simulink model "ModeloManual"  (R2022a)
settings: Solver=VariableStepAuto  StartTime=0.0  StopTime=10  RelTol=1e-3
values from neighbouring files (symbols this model uses):
  a = 0.2    [Data.m]
  alturaobst = 0.9    [Data.m]
  b = 0.542    [Data.m]
  M = [x_new y_new]    [Data.m]
  M_chasis = 3    [Data.m]
  M_rueda = 1    [Data.m]
  M_ruedacontacto = 1    [Data.m]
  N = 4365    [GraficasVelocidades.m]    (also in Prueba_Liapunov.m = length(p_X); WaypointsToTrayectory.m = length(X))
  R = 0.175/2    (= 0.0875)    [Data.m]
  X = M(:,1)    [WaypointsToTrayectory.m]
  x0 = x_ini(1)*factorE    [Data.m]
  x_obj = pos_fin(1)*factorE    [Data.m]
  xobstac = RandomPos(1)    [Data.m]
  Y = M(:, 2)    [WaypointsToTrayectory.m]
  y0 = y_ini(2)*factorE    [Data.m]
  y_obj = pos_fin(2)*factorE    [Data.m]
  yobstac = RandomPos(2)    [Data.m]
  zobstac = RandomPos(3)    [Data.m]
undefined symbols (not defined in the file or in its folder): bloqueobstaculo, Borde11, Borde12, Borde2, Borde3, Borde41, Borde42, Explanada, plano150g1, plano150g2, plano150g3, plano150g4, Plano150mm, plano150mm2irr, Plano45mm, plano45mm2irr, Plano90mm, Rampa, Rampa21, Rampa22, Rampa31, Rampa32, Rampa33, Rampa4, Rampa51, Rampa52, Rampa53, Terreno, Z
libraries: sm_lib x331, nesl_utility x30, fl_lib x3, robotalgslib x1
(part 5 of 8)

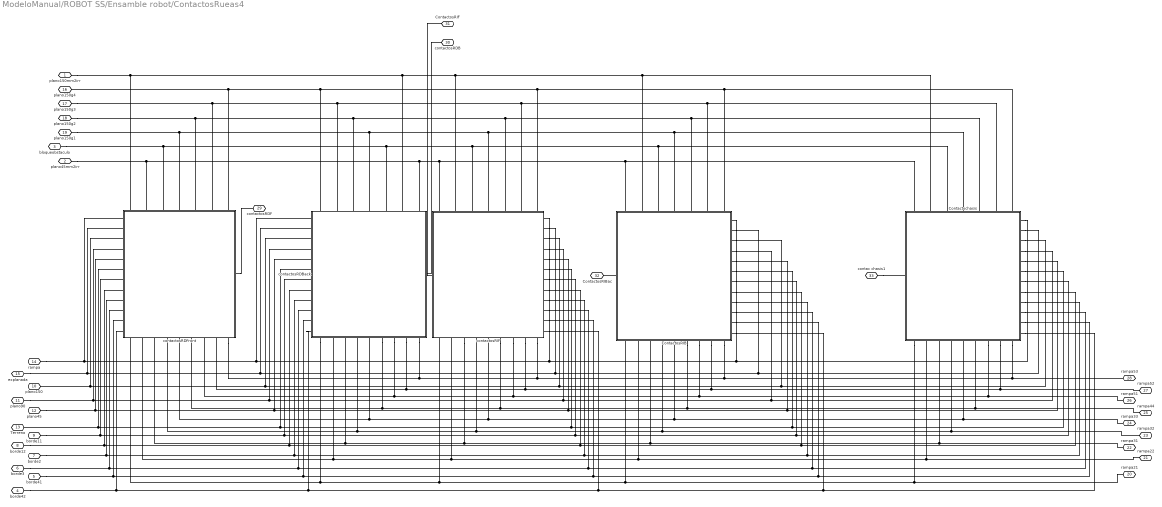
== system ModeloManual/ROBOT SS/Ensamble robot/ContactosRueas4 ==
  Contactochasis : Subsystem
      settings: PortSchema="{\"entries\":[{\"content\":{\"sides\":[{\"content\":{\"connectorIds\":[\"LConn1\"]},\"type\":\"ConnectorPlacement.EquallySpacedRectSide\",\"uuid\":\"4f581815-8ae4-4ee7-9b05-a8dd2e10ae63\"},{\"content\":{\"connectorIds\":[\"RConn1\",\"RConn2\",\"RConn3\",\"RConn4\",\"RConn5\",\"RConn6\",\"RConn7\",\"RConn8\",\"RConn9\",\"RConn10\",\"RConn11\",\"RConn12\"],\"side\":\"RIGHT\"},\"type\":\"ConnectorPlacement.EquallySpacedRectSide\",\"uuid\":\"8325c4e1-14be-4d51-94f3-53093c654f2d\"},{\"content\":{\"connectorIds\":[\"LConn2\",\"LConn3\",\"LConn4\",\"LConn5\",\"LConn6\",\"LConn7\",\"LConn8\",\"LConn9\",\"LConn10\"],\"side\":\"TOP\"},\"type\":\"ConnectorPlacement.EquallySpacedRectSide\",\"uuid\":\"45878acc-deff-4729-a66d-73775d7e8d0b\"},{\"content\":{\"connectorIds\":[\"RConn13\",\"RConn14\",\"RConn15\",\"RConn16\",\"RConn17\",\"RConn18\",\"RConn19\"],\"side\":\"BOTTOM\"},\"type\":\"ConnectorPlacement.EquallySpacedRectSide\",\"uuid\":\"dca1d019-3cd3-4a64-96c4-a5ef2847eb3c\"}]},\"type\":\"ConnectorPlacement.EquallySpacedConnector\",\"uuid\":\"5432a14d-752f-4214-bad7-a9a48797e409\"}],\"packageUris\":[\"http://schema.mathworks.com/mf0/Connector/R2020b\"],\"version\":\"1.0\"}"
  ContactosRIB : Subsystem
      settings: PortSchema="{\"entries\":[{\"content\":{\"sides\":[{\"content\":{\"connectorIds\":[\"LConn1\"]},\"type\":\"ConnectorPlacement.EquallySpacedRectSide\",\"uuid\":\"4f581815-8ae4-4ee7-9b05-a8dd2e10ae63\"},{\"content\":{\"connectorIds\":[\"RConn1\",\"RConn2\",\"RConn3\",\"RConn4\",\"RConn5\",\"RConn6\",\"RConn7\",\"RConn8\",\"RConn9\",\"RConn10\",\"RConn11\",\"RConn12\"],\"side\":\"RIGHT\"},\"type\":\"ConnectorPlacement.EquallySpacedRectSide\",\"uuid\":\"8325c4e1-14be-4d51-94f3-53093c654f2d\"},{\"content\":{\"connectorIds\":[\"LConn2\",\"LConn3\",\"LConn4\",\"LConn5\",\"LConn6\",\"LConn7\",\"LConn8\",\"LConn9\",\"LConn10\"],\"side\":\"TOP\"},\"type\":\"ConnectorPlacement.EquallySpacedRectSide\",\"uuid\":\"45878acc-deff-4729-a66d-73775d7e8d0b\"},{\"content\":{\"connectorIds\":[\"RConn13\",\"RConn14\",\"RConn15\",\"RConn16\",\"RConn17\",\"RConn18\",\"RConn19\"],\"side\":\"BOTTOM\"},\"type\":\"ConnectorPlacement.EquallySpacedRectSide\",\"uuid\":\"dca1d019-3cd3-4a64-96c4-a5ef2847eb3c\"}]},\"type\":\"ConnectorPlacement.EquallySpacedConnector\",\"uuid\":\"5432a14d-752f-4214-bad7-a9a48797e409\"}],\"packageUris\":[\"http://schema.mathworks.com/mf0/Connector/R2020b\"],\"version\":\"1.0\"}"
  contactosRDBack : Subsystem
      settings: PortSchema="{\"entries\":[{\"content\":{\"sides\":[{\"content\":{\"connectorIds\":[\"LConn1\",\"LConn2\",\"LConn3\",\"LConn4\",\"LConn5\",\"LConn6\",\"LConn7\",\"LConn8\",\"LConn9\",\"LConn10\",\"LConn11\",\"LConn12\"]},\"type\":\"ConnectorPlacement.EquallySpacedRectSide\",\"uuid\":\"4677d3c0-fe6b-4e84-8f73-c854d9b35b96\"},{\"content\":{\"connectorIds\":[\"RConn1\"],\"side\":\"RIGHT\"},\"type\":\"ConnectorPlacement.EquallySpacedRectSide\",\"uuid\":\"c55e0516-1ae0-4a26-a435-c2ac17281f56\"},{\"content\":{\"connectorIds\":[\"LConn13\",\"LConn14\",\"LConn15\",\"LConn16\",\"LConn17\",\"LConn18\",\"LConn19\",\"LConn20\",\"LConn21\"],\"side\":\"TOP\"},\"type\":\"ConnectorPlacement.EquallySpacedRectSide\",\"uuid\":\"54ab0c51-bb18-4865-8b25-0e77e88e8b63\"},{\"content\":{\"connectorIds\":[\"RConn2\",\"RConn3\",\"RConn4\",\"RConn5\",\"RConn6\",\"RConn7\",\"RConn8\"],\"side\":\"BOTTOM\"},\"type\":\"ConnectorPlacement.EquallySpacedRectSide\",\"uuid\":\"810dc9ff-bd8f-4485-b930-6348a4343a1c\"}]},\"type\":\"ConnectorPlacement.EquallySpacedConnector\",\"uuid\":\"c5f80127-49af-43c5-b6ef-5a46cea3903d\"}],\"packageUris\":[\"http://schema.mathworks.com/mf0/Connector/R2020b\"],\"version\":\"1.0\"}"
  contactosRDFront : Subsystem
      settings: PortSchema="{\"entries\":[{\"content\":{\"sides\":[{\"content\":{\"connectorIds\":[\"LConn1\",\"LConn2\",\"LConn3\",\"LConn4\",\"LConn5\",\"LConn6\",\"LConn7\",\"LConn8\",\"LConn9\",\"LConn10\",\"LConn11\",\"LConn12\"]},\"type\":\"ConnectorPlacement.EquallySpacedRectSide\",\"uuid\":\"4677d3c0-fe6b-4e84-8f73-c854d9b35b96\"},{\"content\":{\"connectorIds\":[\"RConn1\"],\"side\":\"RIGHT\"},\"type\":\"ConnectorPlacement.EquallySpacedRectSide\",\"uuid\":\"c55e0516-1ae0-4a26-a435-c2ac17281f56\"},{\"content\":{\"connectorIds\":[\"LConn13\",\"LConn14\",\"LConn15\",\"LConn16\",\"LConn17\",\"LConn18\",\"LConn19\",\"LConn20\",\"LConn21\"],\"side\":\"TOP\"},\"type\":\"ConnectorPlacement.EquallySpacedRectSide\",\"uuid\":\"54ab0c51-bb18-4865-8b25-0e77e88e8b63\"},{\"content\":{\"connectorIds\":[\"RConn2\",\"RConn3\",\"RConn4\",\"RConn5\",\"RConn6\",\"RConn7\",\"RConn8\"],\"side\":\"BOTTOM\"},\"type\":\"ConnectorPlacement.EquallySpacedRectSide\",\"uuid\":\"1e9ef993-c1dc-4ae7-9992-9b6ea278c652\"}]},\"type\":\"ConnectorPlacement.EquallySpacedConnector\",\"uuid\":\"c5f80127-49af-43c5-b6ef-5a46cea3903d\"}],\"packageUris\":[\"http://schema.mathworks.com/mf0/Connector/R2020b\"],\"version\":\"1.0\"}"
  contactosRIF : Subsystem
      settings: PortSchema="{\"entries\":[{\"content\":{\"sides\":[{\"content\":{\"connectorIds\":[\"LConn1\"]},\"type\":\"ConnectorPlacement.EquallySpacedRectSide\",\"uuid\":\"4f581815-8ae4-4ee7-9b05-a8dd2e10ae63\"},{\"content\":{\"connectorIds\":[\"RConn1\",\"RConn2\",\"RConn3\",\"RConn4\",\"RConn5\",\"RConn6\",\"RConn7\",\"RConn8\",\"RConn9\",\"RConn10\",\"RConn11\",\"RConn12\"],\"side\":\"RIGHT\"},\"type\":\"ConnectorPlacement.EquallySpacedRectSide\",\"uuid\":\"8325c4e1-14be-4d51-94f3-53093c654f2d\"},{\"content\":{\"connectorIds\":[\"LConn2\",\"LConn3\",\"LConn4\",\"LConn5\",\"LConn6\",\"LConn7\",\"LConn8\",\"LConn9\",\"LConn10\"],\"side\":\"TOP\"},\"type\":\"ConnectorPlacement.EquallySpacedRectSide\",\"uuid\":\"45878acc-deff-4729-a66d-73775d7e8d0b\"},{\"content\":{\"connectorIds\":[\"RConn13\",\"RConn14\",\"RConn15\",\"RConn16\",\"RConn17\",\"RConn18\",\"RConn19\"],\"side\":\"BOTTOM\"},\"type\":\"ConnectorPlacement.EquallySpacedRectSide\",\"uuid\":\"4d447f89-609c-4778-adb6-6019672adf15\"}]},\"type\":\"ConnectorPlacement.EquallySpacedConnector\",\"uuid\":\"5432a14d-752f-4214-bad7-a9a48797e409\"}],\"packageUris\":[\"http://schema.mathworks.com/mf0/Connector/R2020b\"],\"version\":\"1.0\"}"
  plano150mm2irr : PMIOPort  Side=Left
  plano45mm2irr : PMIOPort  Port=2  Side=Left
  bloqueobstaculo : PMIOPort  Port=3  Side=Left
  borde42 : PMIOPort  Port=4  Side=Left
  borde41 : PMIOPort  Port=5  Side=Left
  borde3 : PMIOPort  Port=6  Side=Left
  borde2 : PMIOPort  Port=7  Side=Left
  borde12 : PMIOPort  Port=8  Side=Left
  borde11 : PMIOPort  Port=9  Side=Left
  plano150 : PMIOPort  Port=10  Side=Left
  plano90 : PMIOPort  Port=11  Side=Left
  plano45 : PMIOPort  Port=12  Side=Left
  Terreno : PMIOPort  Port=13  Side=Left
  rampa : PMIOPort  Port=14  Side=Left
  explanada : PMIOPort  Port=15  Side=Left
  plano150g4 : PMIOPort  Port=16  Side=Left
  plano150g3 : PMIOPort  Port=17  Side=Left
  plano150g2 : PMIOPort  Port=18  Side=Left
  plano150g1 : PMIOPort  Port=19  Side=Left
  rampa21 : PMIOPort  Port=20  Side=Left
  rampa22 : PMIOPort  Port=21  Side=Left
  rampa31 : PMIOPort  Port=22  Side=Left
  rampa32 : PMIOPort  Port=23  Side=Left
  rampa33 : PMIOPort  Port=24  Side=Left
  rampa44 : PMIOPort  Port=25  Side=Left
  rampa51 : PMIOPort  Port=26  Side=Left
  rampa52 : PMIOPort  Port=27  Side=Left
  rampa53 : PMIOPort  Port=28  Side=Left
  contactosRDF : PMIOPort  Port=29  Side=Right
  contactosRDB : PMIOPort  Port=30  Side=Right
  ContactosRIF : PMIOPort  Port=31  Side=Right
  ContactosRIBac : PMIOPort  Port=32  Side=Right
  contac chasis1 : PMIOPort  Port=33  Side=Right
  connections:
  plano45/RConn1 -- Contactochasis/RConn8 -- ContactosRIB/RConn8 -- contactosRIF/RConn8 -- contactosRDBack/LConn8 -- contactosRDFront/LConn8
  contactosRDFront/LConn7 -- Contactochasis/RConn7 -- ContactosRIB/RConn7 -- contactosRIF/RConn7 -- contactosRDBack/LConn7 -- Terreno/RConn1
  contactosRDFront/RConn1 -- contactosRDF/RConn1
  contactosRDBack/RConn1 -- contactosRDB/RConn1
  plano90/RConn1 -- Contactochasis/RConn9 -- ContactosRIB/RConn9 -- contactosRIF/RConn9 -- contactosRDBack/LConn9 -- contactosRDFront/LConn9
  explanada/RConn1 -- Contactochasis/RConn11 -- ContactosRIB/RConn11 -- contactosRIF/RConn11 -- contactosRDBack/LConn11 -- contactosRDFront/LConn11
  rampa/RConn1 -- Contactochasis/RConn12 -- ContactosRIB/RConn12 -- contactosRIF/RConn12 -- contactosRDBack/LConn12 -- contactosRDFront/LConn12
  contactosRDFront/LConn10 -- Contactochasis/RConn10 -- ContactosRIB/RConn10 -- contactosRIF/RConn10 -- contactosRDBack/LConn10 -- plano150/RConn1
  ContactosRIF/RConn1 -- contactosRIF/LConn1
  ContactosRIB/LConn1 -- ContactosRIBac/RConn1
  borde11/RConn1 -- Contactochasis/RConn6 -- ContactosRIB/RConn6 -- contactosRIF/RConn6 -- contactosRDBack/LConn6 -- contactosRDFront/LConn6
  borde12/RConn1 -- Contactochasis/RConn5 -- ContactosRIB/RConn5 -- contactosRIF/RConn5 -- contactosRDBack/LConn5 -- contactosRDFront/LConn5
  borde2/RConn1 -- ContactosRIB/RConn4 -- Contactochasis/RConn4 -- contactosRIF/RConn4 -- contactosRDBack/LConn4 -- contactosRDFront/LConn4
  borde3/RConn1 -- Contactochasis/RConn3 -- ContactosRIB/RConn3 -- contactosRIF/RConn3 -- contactosRDBack/LConn3 -- contactosRDFront/LConn3
  borde41/RConn1 -- Contactochasis/RConn2 -- ContactosRIB/RConn2 -- contactosRIF/RConn2 -- contactosRDBack/LConn2 -- contactosRDFront/LConn2
  borde42/RConn1 -- Contactochasis/RConn1 -- ContactosRIB/RConn1 -- contactosRIF/RConn1 -- contactosRDBack/LConn1 -- contactosRDFront/LConn1
  contactosRDFront/LConn21 -- contactosRDBack/LConn21 -- contactosRIF/LConn10 -- ContactosRIB/LConn10 -- rampa53/RConn1 -- Contactochasis/LConn10
  rampa52/RConn1 -- Contactochasis/LConn9 -- ContactosRIB/LConn9 -- contactosRIF/LConn9 -- contactosRDBack/LConn20 -- contactosRDFront/LConn20
  rampa51/RConn1 -- Contactochasis/LConn8 -- ContactosRIB/LConn8 -- contactosRIF/LConn8 -- contactosRDBack/LConn19 -- contactosRDFront/LConn19
  rampa44/RConn1 -- Contactochasis/LConn7 -- ContactosRIB/LConn7 -- contactosRIF/LConn7 -- contactosRDBack/LConn18 -- contactosRDFront/LConn18
  rampa33/RConn1 -- Contactochasis/LConn6 -- ContactosRIB/LConn6 -- contactosRIF/LConn6 -- contactosRDBack/LConn17 -- contactosRDFront/LConn17
  rampa32/RConn1 -- Contactochasis/LConn5 -- ContactosRIB/LConn5 -- contactosRIF/LConn5 -- contactosRDBack/LConn16 -- contactosRDFront/LConn16
  rampa31/RConn1 -- Contactochasis/LConn4 -- ContactosRIB/LConn4 -- contactosRIF/LConn4 -- contactosRDBack/LConn15 -- contactosRDFront/LConn15
  rampa22/RConn1 -- Contactochasis/LConn3 -- ContactosRIB/LConn3 -- contactosRIF/LConn3 -- contactosRDBack/LConn14 -- contactosRDFront/LConn14
  rampa21/RConn1 -- ContactosRIB/LConn2 -- contactosRIF/LConn2 -- contactosRDBack/LConn13 -- contactosRDFront/LConn13 -- Contactochasis/LConn2
  contac chasis1/RConn1 -- Contactochasis/LConn1
  Contactochasis/RConn19 -- contactosRIF/RConn19 -- contactosRDFront/RConn8 -- plano150g4/RConn1 -- contactosRDBack/RConn2 -- ContactosRIB/RConn19
  plano150g3/RConn1 -- contactosRIF/RConn18 -- ContactosRIB/RConn18 -- Contactochasis/RConn18 -- contactosRDBack/RConn3 -- contactosRDFront/RConn7
  plano150g2/RConn1 -- contactosRDFront/RConn6 -- contactosRDBack/RConn4 -- contactosRIF/RConn17 -- Contactochasis/RConn17 -- ContactosRIB/RConn17
  plano150g1/RConn1 -- contactosRIF/RConn16 -- ContactosRIB/RConn16 -- Contactochasis/RConn16 -- contactosRDBack/RConn5 -- contactosRDFront/RConn5
  bloqueobstaculo/RConn1 -- contactosRDBack/RConn6 -- contactosRIF/RConn15 -- ContactosRIB/RConn15 -- Contactochasis/RConn15 -- contactosRDFront/RConn4
  plano150mm2irr/RConn1 -- contactosRIF/RConn14 -- ContactosRIB/RConn14 -- Contactochasis/RConn14 -- contactosRDBack/RConn7 -- contactosRDFront/RConn2
  plano45mm2irr/RConn1 -- ContactosRIB/RConn13 -- Contactochasis/RConn13 -- contactosRIF/RConn13 -- contactosRDBack/RConn8 -- contactosRDFront/RConn3

== system ModeloManual/ROBOT SS/Ensamble robot/RDBack ==
  Cylindrical Solid : sm_lib/Body Elements/Cylindrical Solid  GraphicAmbientColor=[0.15 0.15 0.15 1.0]  BasedOnType=Mass  CenterOfMass=[0 0 0]  CenterOfMassUnits=m  GraphicDiffuseColor=[1.0 0.0 0.2]  CylinderLength=0.045  CylinderLengthUnits=m  CylinderRadius=0.0826  CylinderRadiusUnits=m  Density=1000  DensityUnits=kg/m^3  DoExposeReferenceFrame=on  GraphicEmissiveColor=[0.0 0.0 0.0 1.0]  ExportEntireGeometry=on  SerializedFrames=<Frames/>  MarkerShape=Sphere  MarkerSize=10  GraphicType=None  InertiaType=CalculateFromGeometry  Mass=M_ruedacontacto  MassUnits=kg  MomentsOfInertia=[1 1 1]  MomentsOfInertiaUnits=kg*m^2  GraphicOpacity=1.0  ProductsOfInertia=[0 0 0]  ProductsOfInertiaUnits=kg*m^2  GraphicShininess=75  GraphicSpecularColor=[0.5 0.5 0.5 1.0]  GraphicVisPropType=SimpleVisualProperties
  PS-Simulink Converter : nesl_utility/PS-Simulink Converter  PhysicalDomain=network_engine_domain  SubClassName=ps_output  LeftPortType=input  RightPortType=output  PseudoPeriodic=off  Frequencies=[]  VectorFormat=inherit  Unit=inherit  AffineConversion=off
      settings: SourceProductBaseCode=SS,PW,VE
  Revolute Joint1 : sm_lib/Joints/Revolute Joint  JointMode=Normal  SenseConstraintForce=off  SenseConstraintForceX=off  SenseConstraintForceY=off  SenseConstraintForceZ=off  SenseConstraintTorque=off  SenseConstraintTorqueX=off  SenseConstraintTorqueY=off  SenseConstraintTorqueZ=off  SenseTotalForce=off  SenseTotalForceX=off  SenseTotalForceY=off  SenseTotalForceZ=off  SenseTotalTorque=off  SenseTotalTorqueX=off  SenseTotalTorqueY=off  SenseTotalTorqueZ=off  CompositeWrenchDir=FollowerOnBase  CompositeWrenchFrame=BaseFrame  EquilibriumPosition=0  EquilibriumPositionUnits=rad  SpringStiffness=0  SpringStiffnessUnits=N*m/rad  DampingCoefficient=0  DampingCoefficientUnits=N*m/(rad/s)  TorqueActuationMode=ComputedTorque  MotionActuationMode=InputMotion  SensePosition=off  SenseVelocity=on  SenseAcceleration=off  SenseTorqueForce=off  SenseLowerLimitTorqueForce=off  SenseUpperLimitTorqueForce=off  LowerLimitSpecify=off  LowerLimitBound=-90  LowerLimitBoundUnits=deg  LowerLimitStiffness=1e4  LowerLimitStiffnessUnits=N*m/deg  LowerLimitDamping=10  LowerLimitDampingUnits=N*m/(deg/s)  LowerLimitTransitionRegionWidth=0.1  LowerLimitTransitionRegionWidthUnits=deg  UpperLimitSpecify=off  UpperLimitBound=90  UpperLimitBoundUnits=deg  UpperLimitStiffness=1e4  UpperLimitStiffnessUnits=N*m/deg  UpperLimitDamping=10  UpperLimitDampingUnits=N*m/(deg/s)  UpperLimitTransitionRegionWidth=0.1  UpperLimitTransitionRegionWidthUnits=deg  PositionTargetSpecify=off  PositionTargetPriority=High  PositionTargetValue=0  PositionTargetValueUnits=deg  VelocityTargetSpecify=off  VelocityTargetPriority=High  VelocityTargetValue=0  VelocityTargetValueUnits=deg/s
  Rigid Transform1 : sm_lib/Frames and Transforms/Rigid Transform  TranslationMethod=None  TranslationStandardOffset=10  TranslationLengthUnit=mm  TranslationStandardAxis=-X  TranslationCartesianOffset=[0 0 0]  TranslationROffset=0  TranslationROffsetUnits=m  TranslationZOffset=0  TranslationZOffsetUnits=m  TranslationThetaOffset=0  TranslationThetaOffsetUnits=deg  RotationMethod=StandardAxis  RotationAngleUnits=deg  RotationStandardAxis=-Y  RotationAngle=90  RotationArbitraryAxis=[0 0 1]  FollAlignAxisA=+X  BaseAlignAxisA=+Y  FollAlignAxisB=+Y  BaseAlignAxisB=+Z  RotationSequenceAxes=FollowerAxes  RotationSequence=XYZ  RotationSequenceAngles=[0 0 0]  RotationSequenceAnglesUnits=deg  RotationMatrix=[1 0 0; 0 1 0; 0 0 1]
  Rueda1 : sm_lib/Body Elements/File Solid  ExtGeomFileName=rueda_nueva_contodo.stp  UnitType=FromFile  ExtGeomFileUnits=m  StepReaderType=HEX  ExportConvexHullGeometry=off  InertiaType=CalculateFromGeometry  Mass=M_rueda  MassUnits=kg  CenterOfMass=[0 0 0]  CenterOfMassUnits=m  MomentsOfInertia=[1 1 1]  MomentsOfInertiaUnits=kg*m^2  ProductsOfInertia=[0 0 0]  ProductsOfInertiaUnits=kg*m^2  BasedOnType=Density  Density=D_rueda  DensityUnits=kg/m^3  DoExposeReferenceFrame=on  SerializedFrames=<Frames><Frame><Id>Frame1</Id><Value><Name>F1</Name><Origin><Source>CenterOfMassFrame</Source><FeatureName></FeatureName></Origin><PrimaryAxis><DefinedDirection>+X</DefinedDirection><Source>ReferenceFrame</Source><SourceDirection>+Z</SourceDirection><FeatureName></FeatureName></PrimaryAxis><SecondaryAxis><DefinedDirection>-Z</DefinedDirection><Source>ReferenceFrame</Source><SourceDirection>+X</SourceDirection><FeatureName></FeatureName></SecondaryAxis></Value></Frame></Frames>  GraphicType=FromGeometry  MarkerShape=Sphere  MarkerSize=10  GraphicVisPropType=SimpleVisualProperties  GraphicDiffuseColor=[0 0 0]  GraphicSpecularColor=[0.5 0.5 0.5 1.0]  GraphicAmbientColor=[0.15 0.15 0.15 1.0]  GraphicEmissiveColor=[0.0 0.0 0.0 1.0]  GraphicShininess=75  GraphicOpacity=1.0
  W2 : PMIOPort  Side=Left
  F : PMIOPort  Port=2  Side=Right
  contactosRDB : PMIOPort  Port=3  Side=Left
  ws : Outport
  wires:
  PS-Simulink Converter/1 -> ws/1
  connections:
  W2/RConn1 -- Revolute Joint1/LConn2
  Revolute Joint1/RConn1 -- F/RConn1
  Rigid Transform1/RConn1 -- Revolute Joint1/LConn1
  Rueda1/RConn1 -- Rigid Transform1/LConn1
  PS-Simulink Converter/LConn1 -- Revolute Joint1/RConn2
  Cylindrical Solid/RConn1 -- Rueda1/LConn1
  Cylindrical Solid/LConn1 -- contactosRDB/RConn1

== system ModeloManual/ROBOT SS/Ensamble robot/RDFront ==
  note: Edificios
  note: Terreno de contacto
  Aulas FIMCP : sm_lib/Body Elements/File Solid  Commented=on  ExtGeomFileName=Edificios\AulasFIMCP.stl  UnitType=Custom  ExtGeomFileUnits=m  StepReaderType=HEX  ExportConvexHullGeometry=off  InertiaType=PointMass  Mass=1000  MassUnits=kg  CenterOfMass=[0 0 0]  CenterOfMassUnits=m  MomentsOfInertia=[1 1 1]  MomentsOfInertiaUnits=kg*m^2  ProductsOfInertia=[0 0 0]  ProductsOfInertiaUnits=kg*m^2  BasedOnType=DensityFromFile  Density=1000  DensityUnits=kg/m^3  DoExposeReferenceFrame=on  SerializedFrames=<Frames/>  GraphicType=FromGeometry  MarkerShape=Sphere  MarkerSize=10  GraphicVisPropType=SimpleVisualProperties  GraphicDiffuseColor=[0.0 0.0 1.0]  GraphicSpecularColor=[0.5 0.5 0.5 1.0]  GraphicAmbientColor=[0.15 0.15 0.15 1.0]  GraphicEmissiveColor=[0.0 0.0 0.0 1.0]  GraphicShininess=75  GraphicOpacity=1.0
  Bloque de contacto : sm_lib/Body Elements/Cylindrical Solid  GraphicAmbientColor=[0.15 0.15 0.15 1.0]  BasedOnType=Density  CenterOfMass=[0 0 0]  CenterOfMassUnits=m  GraphicDiffuseColor=[1.0 0.0 0.2]  CylinderLength=0.045  CylinderLengthUnits=m  CylinderRadius=0.0826  CylinderRadiusUnits=m  Density=D_ruedacontacto  DensityUnits=kg/m^3  DoExposeReferenceFrame=on  GraphicEmissiveColor=[0.0 0.0 0.0 1.0]  ExportEntireGeometry=on  SerializedFrames=<Frames/>  MarkerShape=Sphere  MarkerSize=10  GraphicType=None  InertiaType=CalculateFromGeometry  Mass=M_ruedacontacto  MassUnits=kg  MomentsOfInertia=[1 1 1]  MomentsOfInertiaUnits=kg*m^2  GraphicOpacity=1.0  ProductsOfInertia=[0 0 0]  ProductsOfInertiaUnits=kg*m^2  GraphicShininess=75  GraphicSpecularColor=[0.5 0.5 0.5 1.0]  GraphicVisPropType=SimpleVisualProperties
  Contact Force : sm_lib/Forces and Torques/Spatial Contact Force  Commented=on  SenseContactBaseRotation=off  SenseContactBaseTranslation=off  CoefficientOfDynamicFriction=0.3  CoefficientOfStaticFriction=0.5  NormalDamping=1e3  NormalDampingUnits=N/(m/s)  SenseContactSignal=off  NormalStiffness=1e6  NormalStiffnessUnits=N/m  FrictionalCriticalVelocity=1e-3  FrictionalCriticalVelocityUnits=m/s  ZeroCrossDetectContactStartAndEnd=off  SenseContactFollowerRotation=off  SenseContactFollowerTranslation=off  FrictionType=SmoothStickSlip  SenseFrictionalForceMagnitude=off  SenseNormalForceMagnitude=off  NormalForceType=SmoothSpringDamper  SenseNormalVelocity=off  SenseSeparationDistance=off  SenseTangentialVelocity=off  NormalTransitionRegionWidth=1e-4  NormalTransitionRegionWidthUnits=m
  DecanatoFIMCP : sm_lib/Body Elements/File Solid  Commented=on  ExtGeomFileName=Edificios\LDecanatoFIMCP.stl  UnitType=Custom  ExtGeomFileUnits=m  StepReaderType=HEX  ExportConvexHullGeometry=off  InertiaType=PointMass  Mass=1000  MassUnits=kg  CenterOfMass=[0 0 0]  CenterOfMassUnits=m  MomentsOfInertia=[1 1 1]  MomentsOfInertiaUnits=kg*m^2  ProductsOfInertia=[0 0 0]  ProductsOfInertiaUnits=kg*m^2  BasedOnType=DensityFromFile  Density=1000  DensityUnits=kg/m^3  DoExposeReferenceFrame=on  SerializedFrames=<Frames/>  GraphicType=FromGeometry  MarkerShape=Sphere  MarkerSize=10  GraphicVisPropType=SimpleVisualProperties  GraphicDiffuseColor=[0.0 0.0 1.0]  GraphicSpecularColor=[0.5 0.5 0.5 1.0]  GraphicAmbientColor=[0.15 0.15 0.15 1.0]  GraphicEmissiveColor=[0.0 0.0 0.0 1.0]  GraphicShininess=75  GraphicOpacity=1.0
  FIEC : sm_lib/Body Elements/File Solid  Commented=on  ExtGeomFileName=Edificios\LabFiec_FiecVieja.stl  UnitType=Custom  ExtGeomFileUnits=m  StepReaderType=HEX  ExportConvexHullGeometry=off  InertiaType=PointMass  Mass=100  MassUnits=kg  CenterOfMass=[0 0 0]  CenterOfMassUnits=m  MomentsOfInertia=[1 1 1]  MomentsOfInertiaUnits=kg*m^2  ProductsOfInertia=[0 0 0]  ProductsOfInertiaUnits=kg*m^2  BasedOnType=DensityFromFile  Density=1000  DensityUnits=kg/m^3  DoExposeReferenceFrame=on  SerializedFrames=<Frames/>  GraphicType=FromGeometry  MarkerShape=Sphere  MarkerSize=10  GraphicVisPropType=SimpleVisualProperties  GraphicDiffuseColor=[0.8 0.2 0.0]  GraphicSpecularColor=[0.5 0.5 0.5 1.0]  GraphicAmbientColor=[0.15 0.15 0.15 1.0]  GraphicEmissiveColor=[0.0 0.0 0.0 1.0]  GraphicShininess=75  GraphicOpacity=1.0
  Floor : sm_lib/Curves and Surfaces/Infinite Plane  Commented=on  GraphicType=Rectangle  GraphicPlaneWidth=1600  GraphicPlaneWidthUnits=m  GraphicPlaneHeight=1000  GraphicPlaneHeightUnits=m  GraphicVisPropType=SimpleVisualProperties  GraphicDiffuseColor=[0.8 0.8 0.8]  GraphicOpacity=1  GraphicSpecularColor=[0.5 0.5 0.5 1.0]  GraphicAmbientColor=[0.15 0.15 0.15 1.0]  GraphicEmissiveColor=[0.0 0.0 0.0 1.0]  GraphicShininess=75
  Oficinas FIEC : sm_lib/Body Elements/File Solid  Commented=on  ExtGeomFileName=Edificios\oficinaFiec.stl  UnitType=Custom  ExtGeomFileUnits=m  StepReaderType=HEX  ExportConvexHullGeometry=off  InertiaType=PointMass  Mass=100  MassUnits=kg  CenterOfMass=[0 0 0]  CenterOfMassUnits=m  MomentsOfInertia=[1 1 1]  MomentsOfInertiaUnits=kg*m^2  ProductsOfInertia=[0 0 0]  ProductsOfInertiaUnits=kg*m^2  BasedOnType=DensityFromFile  Density=1000  DensityUnits=kg/m^3  DoExposeReferenceFrame=on  SerializedFrames=<Frames/>  GraphicType=FromGeometry  MarkerShape=Sphere  MarkerSize=10  GraphicVisPropType=SimpleVisualProperties  GraphicDiffuseColor=[0.8 0.2 0]  GraphicSpecularColor=[0.5 0.5 0.5 1.0]  GraphicAmbientColor=[0.15 0.15 0.15 1.0]  GraphicEmissiveColor=[0.0 0.0 0.0 1.0]  GraphicShininess=75  GraphicOpacity=1.0
  PS-Simulink Converter : nesl_utility/PS-Simulink Converter  PhysicalDomain=network_engine_domain  SubClassName=ps_output  LeftPortType=input  RightPortType=output  PseudoPeriodic=off  Frequencies=[]  VectorFormat=inherit  Unit=inherit  AffineConversion=off
      settings: SourceProductBaseCode=SS,PW,VE
  Patio de comida : sm_lib/Body Elements/File Solid  Commented=on  ExtGeomFileName=Edificios\patiodecomida.stl  UnitType=Custom  ExtGeomFileUnits=m  StepReaderType=HEX  ExportConvexHullGeometry=off  InertiaType=PointMass  Mass=1000  MassUnits=kg  CenterOfMass=[0 0 0]  CenterOfMassUnits=m  MomentsOfInertia=[1 1 1]  MomentsOfInertiaUnits=kg*m^2  ProductsOfInertia=[0 0 0]  ProductsOfInertiaUnits=kg*m^2  BasedOnType=DensityFromFile  Density=1000  DensityUnits=kg/m^3  DoExposeReferenceFrame=on  SerializedFrames=<Frames/>  GraphicType=FromGeometry  MarkerShape=Sphere  MarkerSize=10  GraphicVisPropType=SimpleVisualProperties  GraphicDiffuseColor=[1.0 1.0 0.0]  GraphicSpecularColor=[0.5 0.5 0.5 1.0]  GraphicAmbientColor=[0.15 0.15 0.15 1.0]  GraphicEmissiveColor=[0.0 0.0 0.0 1.0]  GraphicShininess=75  GraphicOpacity=1.0
  Revolute Joint : sm_lib/Joints/Revolute Joint  JointMode=Normal  SenseConstraintForce=off  SenseConstraintForceX=off  SenseConstraintForceY=off  SenseConstraintForceZ=off  SenseConstraintTorque=off  SenseConstraintTorqueX=off  SenseConstraintTorqueY=off  SenseConstraintTorqueZ=off  SenseTotalForce=off  SenseTotalForceX=off  SenseTotalForceY=off  SenseTotalForceZ=off  SenseTotalTorque=off  SenseTotalTorqueX=off  SenseTotalTorqueY=off  SenseTotalTorqueZ=off  CompositeWrenchDir=FollowerOnBase  CompositeWrenchFrame=BaseFrame  EquilibriumPosition=0  EquilibriumPositionUnits=rad  SpringStiffness=0  SpringStiffnessUnits=N*m/rad  DampingCoefficient=0  DampingCoefficientUnits=N*m/(rad/s)  TorqueActuationMode=ComputedTorque  MotionActuationMode=InputMotion  SensePosition=off  SenseVelocity=on  SenseAcceleration=off  SenseTorqueForce=off  SenseLowerLimitTorqueForce=off  SenseUpperLimitTorqueForce=off  LowerLimitSpecify=off  LowerLimitBound=-90  LowerLimitBoundUnits=deg  LowerLimitStiffness=1e4  LowerLimitStiffnessUnits=N*m/deg  LowerLimitDamping=10  LowerLimitDampingUnits=N*m/(deg/s)  LowerLimitTransitionRegionWidth=0.1  LowerLimitTransitionRegionWidthUnits=deg  UpperLimitSpecify=off  UpperLimitBound=90  UpperLimitBoundUnits=deg  UpperLimitStiffness=1e4  UpperLimitStiffnessUnits=N*m/deg  UpperLimitDamping=10  UpperLimitDampingUnits=N*m/(deg/s)  UpperLimitTransitionRegionWidth=0.1  UpperLimitTransitionRegionWidthUnits=deg  PositionTargetSpecify=off  PositionTargetPriority=High  PositionTargetValue=0  PositionTargetValueUnits=deg  VelocityTargetSpecify=off  VelocityTargetPriority=High  VelocityTargetValue=0  VelocityTargetValueUnits=deg/s
  Rigid Transform : sm_lib/Frames and Transforms/Rigid Transform  TranslationMethod=None  TranslationStandardOffset=10  TranslationLengthUnit=mm  TranslationStandardAxis=-X  TranslationCartesianOffset=[0 0 0]  TranslationROffset=0  TranslationROffsetUnits=m  TranslationZOffset=0  TranslationZOffsetUnits=m  TranslationThetaOffset=0  TranslationThetaOffsetUnits=deg  RotationMethod=StandardAxis  RotationAngleUnits=deg  RotationStandardAxis=-Y  RotationAngle=90  RotationArbitraryAxis=[0 0 1]  FollAlignAxisA=+X  BaseAlignAxisA=+Y  FollAlignAxisB=+Y  BaseAlignAxisB=+Z  RotationSequenceAxes=FollowerAxes  RotationSequence=XYZ  RotationSequenceAngles=[0 0 0]  RotationSequenceAnglesUnits=deg  RotationMatrix=[1 0 0; 0 1 0; 0 0 1]
  Rigid Transform1 : sm_lib/Frames and Transforms/Rigid Transform  Commented=on  TranslationMethod=Cartesian  TranslationStandardOffset=0  TranslationLengthUnit=m  TranslationStandardAxis=+Z  TranslationCartesianOffset=[-160 -250 0]  TranslationROffset=0  TranslationROffsetUnits=m  TranslationZOffset=0  TranslationZOffsetUnits=m  TranslationThetaOffset=0  TranslationThetaOffsetUnits=deg  RotationMethod=StandardAxis  RotationAngleUnits=deg  RotationStandardAxis=+Z  RotationAngle=0  RotationArbitraryAxis=[0 0 1]  FollAlignAxisA=+X  BaseAlignAxisA=+Y  FollAlignAxisB=+Y  BaseAlignAxisB=+Z  RotationSequenceAxes=FollowerAxes  RotationSequence=XYX  RotationSequenceAngles=[0 0 0]  RotationSequenceAnglesUnits=deg  RotationMatrix=[1 0 0; 0 1 0; 0 0 1]
  Rigid Transform10 : sm_lib/Frames and Transforms/Rigid Transform  Commented=on  TranslationMethod=Cartesian  TranslationStandardOffset=0  TranslationLengthUnit=m  TranslationStandardAxis=+Z  TranslationCartesianOffset=[-160 -249.5 0]  TranslationROffset=0  TranslationROffsetUnits=m  TranslationZOffset=0  TranslationZOffsetUnits=m  TranslationThetaOffset=0  TranslationThetaOffsetUnits=deg  RotationMethod=StandardAxis  RotationAngleUnits=deg  RotationStandardAxis=+Z  RotationAngle=0  RotationArbitraryAxis=[0 0 1]  FollAlignAxisA=+X  BaseAlignAxisA=+Y  FollAlignAxisB=+Y  BaseAlignAxisB=+Z  RotationSequenceAxes=FollowerAxes  RotationSequence=XYX  RotationSequenceAngles=[0 0 0]  RotationSequenceAnglesUnits=deg  RotationMatrix=[1 0 0; 0 1 0; 0 0 1]
  Rigid Transform11 : sm_lib/Frames and Transforms/Rigid Transform  Commented=on  TranslationMethod=Cartesian  TranslationStandardOffset=0  TranslationLengthUnit=m  TranslationStandardAxis=+Z  TranslationCartesianOffset=[-215 -240 0]  TranslationROffset=0  TranslationROffsetUnits=m  TranslationZOffset=0  TranslationZOffsetUnits=m  TranslationThetaOffset=0  TranslationThetaOffsetUnits=deg  RotationMethod=StandardAxis  RotationAngleUnits=deg  RotationStandardAxis=+Z  RotationAngle=0  RotationArbitraryAxis=[0 0 1]  FollAlignAxisA=+X  BaseAlignAxisA=+Y  FollAlignAxisB=+Y  BaseAlignAxisB=+Z  RotationSequenceAxes=FollowerAxes  RotationSequence=XYX  RotationSequenceAngles=[0 0 0]  RotationSequenceAnglesUnits=deg  RotationMatrix=[1 0 0; 0 1 0; 0 0 1]
  Rigid Transform13 : sm_lib/Frames and Transforms/Rigid Transform  Commented=on  TranslationMethod=Cartesian  TranslationStandardOffset=0  TranslationLengthUnit=m  TranslationStandardAxis=+Z  TranslationCartesianOffset=[-196 -180 0]  TranslationROffset=0  TranslationROffsetUnits=m  TranslationZOffset=0  TranslationZOffsetUnits=m  TranslationThetaOffset=0  TranslationThetaOffsetUnits=deg  RotationMethod=StandardAxis  RotationAngleUnits=deg  RotationStandardAxis=+Z  RotationAngle=0  RotationArbitraryAxis=[0 0 1]  FollAlignAxisA=+X  BaseAlignAxisA=+Y  FollAlignAxisB=+Y  BaseAlignAxisB=+Z  RotationSequenceAxes=FollowerAxes  RotationSequence=XYX  RotationSequenceAngles=[0 0 0]  RotationSequenceAnglesUnits=deg  RotationMatrix=[1 0 0; 0 1 0; 0 0 1]
  Rigid Transform8 : sm_lib/Frames and Transforms/Rigid Transform  Commented=on  TranslationMethod=Cartesian  TranslationStandardOffset=0  TranslationLengthUnit=m  TranslationStandardAxis=+Z  TranslationCartesianOffset=[-140 -250 0]  TranslationROffset=0  TranslationROffsetUnits=m  TranslationZOffset=0  TranslationZOffsetUnits=m  TranslationThetaOffset=0  TranslationThetaOffsetUnits=deg  RotationMethod=StandardAxis  RotationAngleUnits=deg  RotationStandardAxis=+Z  RotationAngle=0  RotationArbitraryAxis=[0 0 1]  FollAlignAxisA=+X  BaseAlignAxisA=+Y  FollAlignAxisB=+Y  BaseAlignAxisB=+Z  RotationSequenceAxes=FollowerAxes  RotationSequence=XYX  RotationSequenceAngles=[0 0 0]  RotationSequenceAnglesUnits=deg  RotationMatrix=[1 0 0; 0 1 0; 0 0 1]
  Rigid Transform9 : sm_lib/Frames and Transforms/Rigid Transform  Commented=on  TranslationMethod=Cartesian  TranslationStandardOffset=0  TranslationLengthUnit=m  TranslationStandardAxis=+Z  TranslationCartesianOffset=[-155 -250 0]  TranslationROffset=0  TranslationROffsetUnits=m  TranslationZOffset=0  TranslationZOffsetUnits=m  TranslationThetaOffset=0  TranslationThetaOffsetUnits=deg  RotationMethod=StandardAxis  RotationAngleUnits=deg  RotationStandardAxis=+Z  RotationAngle=0  RotationArbitraryAxis=[0 0 1]  FollAlignAxisA=+X  BaseAlignAxisA=+Y  FollAlignAxisB=+Y  BaseAlignAxisB=+Z  RotationSequenceAxes=FollowerAxes  RotationSequence=XYX  RotationSequenceAngles=[0 0 0]  RotationSequenceAnglesUnits=deg  RotationMatrix=[1 0 0; 0 1 0; 0 0 1]
  Rueda : sm_lib/Body Elements/File Solid  ExtGeomFileName=rueda_nueva_contodo.stp  UnitType=FromFile  ExtGeomFileUnits=m  StepReaderType=HEX  ExportConvexHullGeometry=off  InertiaType=CalculateFromGeometry  Mass=M_rueda  MassUnits=kg  CenterOfMass=[0 0 0]  CenterOfMassUnits=m  MomentsOfInertia=[1 1 1]  MomentsOfInertiaUnits=kg*m^2  ProductsOfInertia=[0 0 0]  ProductsOfInertiaUnits=kg*m^2  BasedOnType=Density  Density=D_rueda  DensityUnits=kg/m^3  DoExposeReferenceFrame=on  SerializedFrames=<Frames><Frame><Id>Frame1</Id><Value><Name>F1</Name><Origin><Source>CenterOfMassFrame</Source><FeatureName></FeatureName></Origin><PrimaryAxis><DefinedDirection>+X</DefinedDirection><Source>ReferenceFrame</Source><SourceDirection>+Z</SourceDirection><FeatureName></FeatureName></PrimaryAxis><SecondaryAxis><DefinedDirection>-Z</DefinedDirection><Source>ReferenceFrame</Source><SourceDirection>+X</SourceDirection><FeatureName></FeatureName></SecondaryAxis></Value></Frame></Frames>  GraphicType=FromGeometry  MarkerShape=Sphere  MarkerSize=10  GraphicVisPropType=SimpleVisualProperties  GraphicDiffuseColor=[0 0 0]  GraphicSpecularColor=[0.5 0.5 0.5 1.0]  GraphicAmbientColor=[0.15 0.15 0.15 1.0]  GraphicEmissiveColor=[0.0 0.0 0.0 1.0]  GraphicShininess=75  GraphicOpacity=1.0
  Sweet&Coffee : sm_lib/Body Elements/File Solid  Commented=on  ExtGeomFileName=Edificios\sweet.stl  UnitType=Custom  ExtGeomFileUnits=m  StepReaderType=HEX  ExportConvexHullGeometry=off  InertiaType=PointMass  Mass=100  MassUnits=kg  CenterOfMass=[0 0 0]  CenterOfMassUnits=m  MomentsOfInertia=[1 1 1]  MomentsOfInertiaUnits=kg*m^2  ProductsOfInertia=[0 0 0]  ProductsOfInertiaUnits=kg*m^2  BasedOnType=DensityFromFile  Density=1000  DensityUnits=kg/m^3  DoExposeReferenceFrame=on  SerializedFrames=<Frames/>  GraphicType=FromGeometry  MarkerShape=Sphere  MarkerSize=10  GraphicVisPropType=SimpleVisualProperties  GraphicDiffuseColor=[0.0 0.4 0.2]  GraphicSpecularColor=[0.5 0.5 0.5 1.0]  GraphicAmbientColor=[0.15 0.15 0.15 1.0]  GraphicEmissiveColor=[0.0 0.0 0.0 1.0]  GraphicShininess=75  GraphicOpacity=1.0
  W1 : PMIOPort  Side=Left
  F : PMIOPort  Port=2  Side=Right
  contactosRDF : PMIOPort  Port=3  Side=Left
  ws : Outport
  wires:
  PS-Simulink Converter/1 -> ws/1
  connections:
  W1/RConn1 -- Revolute Joint/LConn2
  F/RConn1 -- Revolute Joint/RConn1
  Rigid Transform/RConn1 -- Revolute Joint/LConn1
  PS-Simulink Converter/LConn1 -- Revolute Joint/RConn2
  Rueda/LConn1 -- Bloque de contacto/RConn1
  Rigid Transform/LConn1 -- Rueda/RConn1
  Rigid Transform8/RConn1 -- Rigid Transform10/RConn1 -- Rigid Transform13/RConn1 -- Rigid Transform9/RConn1 -- Rigid Transform1/RConn1 -- Floor/LConn1 -- Rigid Transform11/RConn1
  Contact Force/RConn1 -- Floor/RConn1
  Contact Force/LConn1 -- contactosRDF/RConn1 -- Bloque de contacto/LConn1
  DecanatoFIMCP/RConn1 -- Rigid Transform11/LConn1
  Oficinas FIEC/RConn1 -- Rigid Transform8/LConn1
  Rigid Transform13/LConn1 -- FIEC/RConn1
  Aulas FIMCP/RConn1 -- Rigid Transform9/LConn1
  Sweet&Coffee/RConn1 -- Rigid Transform1/LConn1
  Rigid Transform10/LConn1 -- Patio de comida/RConn1

== system ModeloManual/ROBOT SS/Ensamble robot/RIBack ==
  Cylindrical Solid : sm_lib/Body Elements/Cylindrical Solid  GraphicAmbientColor=[0.15 0.15 0.15 1.0]  BasedOnType=Density  CenterOfMass=[0 0 0]  CenterOfMassUnits=m  GraphicDiffuseColor=[1.0 0.0 0.2]  CylinderLength=0.045  CylinderLengthUnits=m  CylinderRadius=0.0826  CylinderRadiusUnits=m  Density=D_ruedacontacto  DensityUnits=kg/m^3  DoExposeReferenceFrame=on  GraphicEmissiveColor=[0.0 0.0 0.0 1.0]  ExportEntireGeometry=on  SerializedFrames=<Frames/>  MarkerShape=Sphere  MarkerSize=10  GraphicType=None  InertiaType=CalculateFromGeometry  Mass=M_ruedacontacto  MassUnits=kg  MomentsOfInertia=[1 1 1]  MomentsOfInertiaUnits=kg*m^2  GraphicOpacity=1.0  ProductsOfInertia=[0 0 0]  ProductsOfInertiaUnits=kg*m^2  GraphicShininess=75  GraphicSpecularColor=[0.5 0.5 0.5 1.0]  GraphicVisPropType=SimpleVisualProperties
  PS-Simulink Converter : nesl_utility/PS-Simulink Converter  PhysicalDomain=network_engine_domain  SubClassName=ps_output  LeftPortType=input  RightPortType=output  PseudoPeriodic=off  Frequencies=[]  VectorFormat=inherit  Unit=inherit  AffineConversion=off
      settings: SourceProductBaseCode=SS,PW,VE
  Revolute Joint1 : sm_lib/Joints/Revolute Joint  JointMode=Normal  SenseConstraintForce=off  SenseConstraintForceX=off  SenseConstraintForceY=off  SenseConstraintForceZ=off  SenseConstraintTorque=off  SenseConstraintTorqueX=off  SenseConstraintTorqueY=off  SenseConstraintTorqueZ=off  SenseTotalForce=off  SenseTotalForceX=off  SenseTotalForceY=off  SenseTotalForceZ=off  SenseTotalTorque=off  SenseTotalTorqueX=off  SenseTotalTorqueY=off  SenseTotalTorqueZ=off  CompositeWrenchDir=FollowerOnBase  CompositeWrenchFrame=BaseFrame  EquilibriumPosition=0  EquilibriumPositionUnits=rad  SpringStiffness=0  SpringStiffnessUnits=N*m/rad  DampingCoefficient=0  DampingCoefficientUnits=N*m/(rad/s)  TorqueActuationMode=ComputedTorque  MotionActuationMode=InputMotion  SensePosition=off  SenseVelocity=on  SenseAcceleration=off  SenseTorqueForce=off  SenseLowerLimitTorqueForce=off  SenseUpperLimitTorqueForce=off  LowerLimitSpecify=off  LowerLimitBound=-90  LowerLimitBoundUnits=deg  LowerLimitStiffness=1e4  LowerLimitStiffnessUnits=N*m/deg  LowerLimitDamping=10  LowerLimitDampingUnits=N*m/(deg/s)  LowerLimitTransitionRegionWidth=0.1  LowerLimitTransitionRegionWidthUnits=deg  UpperLimitSpecify=off  UpperLimitBound=90  UpperLimitBoundUnits=deg  UpperLimitStiffness=1e4  UpperLimitStiffnessUnits=N*m/deg  UpperLimitDamping=10  UpperLimitDampingUnits=N*m/(deg/s)  UpperLimitTransitionRegionWidth=0.1  UpperLimitTransitionRegionWidthUnits=deg  PositionTargetSpecify=off  PositionTargetPriority=High  PositionTargetValue=0  PositionTargetValueUnits=deg  VelocityTargetSpecify=off  VelocityTargetPriority=High  VelocityTargetValue=0  VelocityTargetValueUnits=deg/s
  Rigid Transform1 : sm_lib/Frames and Transforms/Rigid Transform  TranslationMethod=None  TranslationStandardOffset=10  TranslationLengthUnit=mm  TranslationStandardAxis=-X  TranslationCartesianOffset=[0 0 0]  TranslationROffset=0  TranslationROffsetUnits=m  TranslationZOffset=0  TranslationZOffsetUnits=m  TranslationThetaOffset=0  TranslationThetaOffsetUnits=deg  RotationMethod=StandardAxis  RotationAngleUnits=deg  RotationStandardAxis=+Y  RotationAngle=90  RotationArbitraryAxis=[0 0 1]  FollAlignAxisA=+X  BaseAlignAxisA=+Y  FollAlignAxisB=+Y  BaseAlignAxisB=+Z  RotationSequenceAxes=FollowerAxes  RotationSequence=XYZ  RotationSequenceAngles=[0 0 0]  RotationSequenceAnglesUnits=deg  RotationMatrix=[1 0 0; 0 1 0; 0 0 1]
  Rueda1 : sm_lib/Body Elements/File Solid  ExtGeomFileName=rueda_nueva_contodo.stp  UnitType=FromFile  ExtGeomFileUnits=m  StepReaderType=HEX  ExportConvexHullGeometry=off  InertiaType=CalculateFromGeometry  Mass=M_rueda  MassUnits=kg  CenterOfMass=[0 0 0]  CenterOfMassUnits=m  MomentsOfInertia=[1 1 1]  MomentsOfInertiaUnits=kg*m^2  ProductsOfInertia=[0 0 0]  ProductsOfInertiaUnits=kg*m^2  BasedOnType=Density  Density=D_rueda  DensityUnits=kg/m^3  DoExposeReferenceFrame=on  SerializedFrames=<Frames><Frame><Id>Frame1</Id><Value><Name>F1</Name><Origin><Source>CenterOfMassFrame</Source><FeatureName></FeatureName></Origin><PrimaryAxis><DefinedDirection>+X</DefinedDirection><Source>ReferenceFrame</Source><SourceDirection>+Z</SourceDirection><FeatureName></FeatureName></PrimaryAxis><SecondaryAxis><DefinedDirection>-Z</DefinedDirection><Source>ReferenceFrame</Source><SourceDirection>+X</SourceDirection><FeatureName></FeatureName></SecondaryAxis></Value></Frame></Frames>  GraphicType=FromGeometry  MarkerShape=Sphere  MarkerSize=10  GraphicVisPropType=SimpleVisualProperties  GraphicDiffuseColor=[0 0 0]  GraphicSpecularColor=[0.5 0.5 0.5 1.0]  GraphicAmbientColor=[0.15 0.15 0.15 1.0]  GraphicEmissiveColor=[0.0 0.0 0.0 1.0]  GraphicShininess=75  GraphicOpacity=1.0
  w4 : PMIOPort  Side=Left
  F : PMIOPort  Port=2  Side=Right
  contactosRIB : PMIOPort  Port=3  Side=Right
  ws : Outport
  wires:
  PS-Simulink Converter/1 -> ws/1
  connections:
  w4/RConn1 -- Revolute Joint1/LConn2
  Revolute Joint1/RConn1 -- F/RConn1
  Rigid Transform1/RConn1 -- Revolute Joint1/LConn1
  Rueda1/RConn1 -- Rigid Transform1/LConn1
  PS-Simulink Converter/LConn1 -- Revolute Joint1/RConn2
  Cylindrical Solid/RConn1 -- Rueda1/LConn1
  Cylindrical Solid/LConn1 -- contactosRIB/RConn1

== system ModeloManual/ROBOT SS/Ensamble robot/RIFront ==
  Cylindrical Solid : sm_lib/Body Elements/Cylindrical Solid  GraphicAmbientColor=[0.15 0.15 0.15 1.0]  BasedOnType=Density  CenterOfMass=[0 0 0]  CenterOfMassUnits=m  GraphicDiffuseColor=[1.0 0.0 0.2]  CylinderLength=0.045  CylinderLengthUnits=m  CylinderRadius=0.0826  CylinderRadiusUnits=m  Density=D_ruedacontacto  DensityUnits=kg/m^3  DoExposeReferenceFrame=on  GraphicEmissiveColor=[0.0 0.0 0.0 1.0]  ExportEntireGeometry=on  SerializedFrames=<Frames/>  MarkerShape=Sphere  MarkerSize=10  GraphicType=None  InertiaType=CalculateFromGeometry  Mass=M_ruedacontacto  MassUnits=kg  MomentsOfInertia=[1 1 1]  MomentsOfInertiaUnits=kg*m^2  GraphicOpacity=1.0  ProductsOfInertia=[0 0 0]  ProductsOfInertiaUnits=kg*m^2  GraphicShininess=75  GraphicSpecularColor=[0.5 0.5 0.5 1.0]  GraphicVisPropType=SimpleVisualProperties
  PS-Simulink Converter : nesl_utility/PS-Simulink Converter  PhysicalDomain=network_engine_domain  SubClassName=ps_output  LeftPortType=input  RightPortType=output  PseudoPeriodic=off  Frequencies=[]  VectorFormat=inherit  Unit=inherit  AffineConversion=off
      settings: SourceProductBaseCode=SS,PW,VE
  Revolute Joint : sm_lib/Joints/Revolute Joint  JointMode=Normal  SenseConstraintForce=off  SenseConstraintForceX=off  SenseConstraintForceY=off  SenseConstraintForceZ=off  SenseConstraintTorque=off  SenseConstraintTorqueX=off  SenseConstraintTorqueY=off  SenseConstraintTorqueZ=off  SenseTotalForce=off  SenseTotalForceX=off  SenseTotalForceY=off  SenseTotalForceZ=off  SenseTotalTorque=off  SenseTotalTorqueX=off  SenseTotalTorqueY=off  SenseTotalTorqueZ=off  CompositeWrenchDir=FollowerOnBase  CompositeWrenchFrame=BaseFrame  EquilibriumPosition=0  EquilibriumPositionUnits=rad  SpringStiffness=0  SpringStiffnessUnits=N*m/rad  DampingCoefficient=0  DampingCoefficientUnits=N*m/(rad/s)  TorqueActuationMode=ComputedTorque  MotionActuationMode=InputMotion  SensePosition=off  SenseVelocity=on  SenseAcceleration=off  SenseTorqueForce=off  SenseLowerLimitTorqueForce=off  SenseUpperLimitTorqueForce=off  LowerLimitSpecify=off  LowerLimitBound=-90  LowerLimitBoundUnits=deg  LowerLimitStiffness=1e4  LowerLimitStiffnessUnits=N*m/deg  LowerLimitDamping=10  LowerLimitDampingUnits=N*m/(deg/s)  LowerLimitTransitionRegionWidth=0.1  LowerLimitTransitionRegionWidthUnits=deg  UpperLimitSpecify=off  UpperLimitBound=90  UpperLimitBoundUnits=deg  UpperLimitStiffness=1e4  UpperLimitStiffnessUnits=N*m/deg  UpperLimitDamping=10  UpperLimitDampingUnits=N*m/(deg/s)  UpperLimitTransitionRegionWidth=0.1  UpperLimitTransitionRegionWidthUnits=deg  PositionTargetSpecify=off  PositionTargetPriority=High  PositionTargetValue=0  PositionTargetValueUnits=deg  VelocityTargetSpecify=off  VelocityTargetPriority=High  VelocityTargetValue=0  VelocityTargetValueUnits=deg/s
  Rigid Transform : sm_lib/Frames and Transforms/Rigid Transform  TranslationMethod=None  TranslationStandardOffset=10  TranslationLengthUnit=mm  TranslationStandardAxis=-X  TranslationCartesianOffset=[0 0 0]  TranslationROffset=0  TranslationROffsetUnits=m  TranslationZOffset=0  TranslationZOffsetUnits=m  TranslationThetaOffset=0  TranslationThetaOffsetUnits=deg  RotationMethod=StandardAxis  RotationAngleUnits=deg  RotationStandardAxis=+Y  RotationAngle=90  RotationArbitraryAxis=[0 0 1]  FollAlignAxisA=+X  BaseAlignAxisA=+Y  FollAlignAxisB=+Y  BaseAlignAxisB=+Z  RotationSequenceAxes=FollowerAxes  RotationSequence=XYZ  RotationSequenceAngles=[0 90 -90]  RotationSequenceAnglesUnits=deg  RotationMatrix=[1 0 0; 0 1 0; 0 0 1]
  Rueda : sm_lib/Body Elements/File Solid  ExtGeomFileName=rueda_nueva_contodo.stp  UnitType=FromFile  ExtGeomFileUnits=m  StepReaderType=HEX  ExportConvexHullGeometry=off  InertiaType=CalculateFromGeometry  Mass=M_rueda  MassUnits=kg  CenterOfMass=[0 0 0]  CenterOfMassUnits=m  MomentsOfInertia=[1 1 1]  MomentsOfInertiaUnits=kg*m^2  ProductsOfInertia=[0 0 0]  ProductsOfInertiaUnits=kg*m^2  BasedOnType=Density  Density=D_rueda  DensityUnits=kg/m^3  DoExposeReferenceFrame=on  SerializedFrames=<Frames><Frame><Id>Frame1</Id><Value><Name>F1</Name><Origin><Source>CenterOfMassFrame</Source><FeatureName></FeatureName></Origin><PrimaryAxis><DefinedDirection>+X</DefinedDirection><Source>ReferenceFrame</Source><SourceDirection>+Z</SourceDirection><FeatureName></FeatureName></PrimaryAxis><SecondaryAxis><DefinedDirection>-Z</DefinedDirection><Source>ReferenceFrame</Source><SourceDirection>+X</SourceDirection><FeatureName></FeatureName></SecondaryAxis></Value></Frame></Frames>  GraphicType=FromGeometry  MarkerShape=Sphere  MarkerSize=10  GraphicVisPropType=SimpleVisualProperties  GraphicDiffuseColor=[0 0 0]  GraphicSpecularColor=[0.5 0.5 0.5 1.0]  GraphicAmbientColor=[0.15 0.15 0.15 1.0]  GraphicEmissiveColor=[0.0 0.0 0.0 1.0]  GraphicShininess=75  GraphicOpacity=1.0
  w3 : PMIOPort  Side=Left
  F : PMIOPort  Port=2  Side=Right
  cotnactosRIF : PMIOPort  Port=3  Side=Right
  ws : Outport
  wires:
  PS-Simulink Converter/1 -> ws/1
  connections:
  w3/RConn1 -- Revolute Joint/LConn2
  F/RConn1 -- Revolute Joint/RConn1
  Rigid Transform/RConn1 -- Revolute Joint/LConn1
  Rueda/LConn1 -- Cylindrical Solid/RConn1
  Rueda/RConn1 -- Rigid Transform/LConn1
  PS-Simulink Converter/LConn1 -- Revolute Joint/RConn2
  cotnactosRIF/RConn1 -- Cylindrical Solid/LConn1
